simulink model "adc_demo"  (Simulink 10.1)
settings: Solver=VariableStepDiscrete  StartTime=0.0  StopTime=1  RelTol=1e-3  EnableMultiTasking=on
libraries: simulink_extras x3
settings Model: Creator=rcheng  LastModifiedBy=juan
settings DataIOCC: LimitDataPoints=on  SignalLoggingSaveFormat=ModelDataLogs
settings OptimizationCC: ExpressionDepthLimit=2147483647  InitFltsAndDblsToZero=on
settings DebuggingCC: SolverPrmCheckMsg=warning  FcnCallInpInsideContextMsg=warning  StateNameClashWarn=warning
settings ConfigComp: CovHtmlReporting=off  CovSFcnEnable=off

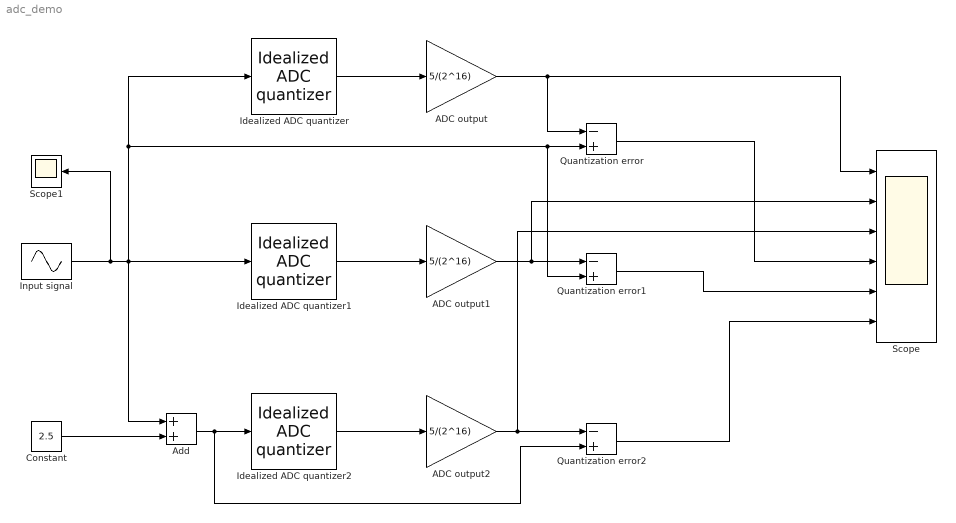
== system adc_demo ==
  ADC output : Gain  Gain=5/(2^16)
  ADC output1 : Gain  Gain=5/(2^16)
  ADC output2 : Gain  Gain=5/(2^16)
  Add : Sum
  Constant : Constant  Value=2.5
  Idealized ADC quantizer : simulink_extras/Additional Discrete/Idealized ADC quantizer  NumberOfConverterBits=16  Vmin=0  Vmax=5  OutputDataType=int16  OutputNegativeValues=on
  Idealized ADC quantizer1 : simulink_extras/Additional Discrete/Idealized ADC quantizer  NumberOfConverterBits=16  Vmin=-2.5  Vmax=2.5  OutputDataType=int16  OutputNegativeValues=on
  Idealized ADC quantizer2 : simulink_extras/Additional Discrete/Idealized ADC quantizer  NumberOfConverterBits=16  Vmin=0  Vmax=5  OutputDataType=uint16  OutputNegativeValues=off
  Input signal : Sin  Amplitude=2.5  Frequency=2*pi*100  SampleTime=1/10000
  Quantization error : Sum  Inputs=-+
  Quantization error1 : Sum  Inputs=-+
  Quantization error2 : Sum  Inputs=-+
  Scope : Scope  NumInputPorts=6
  Scope1 : Scope
  wires:
  Idealized ADC quantizer/1 -> ADC output/1
  ADC output/1 -> Scope/1, Quantization error/1
  Input signal/1 -> Idealized ADC quantizer1/1, Add/1, Quantization error/2, Quantization error1/2, Idealized ADC quantizer/1, Scope1/1
  Idealized ADC quantizer1/1 -> ADC output1/1
  ADC output1/1 -> Scope/2, Quantization error1/1
  Quantization error1/1 -> Scope/5
  Quantization error/1 -> Scope/4
  Idealized ADC quantizer2/1 -> ADC output2/1
  ADC output2/1 -> Scope/3, Quantization error2/1
  Quantization error2/1 -> Scope/6
  Add/1 -> Quantization error2/2, Idealized ADC quantizer2/1
  Constant/1 -> Add/2
